simulink model "etc_ref"  (R2023a)
settings: Solver=ode45  StartTime=0.0  StopTime=20.0  RelTol=1e-3
PreLoadFcn:
  | etc_all_data;
undefined symbols (not defined in the file): J, Ki, Kp, Ts, Vdrop, Vfree, Vopen, Vrise
Description:
  | This is my help
settings Model: ParamWorkspaceSource=ReferencedWorkspace  Creator=nicholas  LastModifiedBy=Administrator
settings SolverCC: AlgebraicLoopSolver=TrustRegion
settings DataIOCC: LimitDataPoints=on  SaveFormat=Array  SignalLoggingSaveFormat=ModelDataLogs  ReturnWorkspaceOutputs=off  SignalLoggingName=sigsOut
settings OptimizationCC: InitFltsAndDblsToZero=on  LifeSpan=inf
settings DebuggingCC: SaveWithParameterizedLinksMsg=none  UnderspecifiedInitializationDetection=Classic  MergeDetectMultiDrivingBlocksExec=none  SignalResolutionControl=TryResolveAllWithWarning  MultiTaskDSMMsg=warning  MultiTaskCondExecSysMsg=none  FcnCallInpInsideContextMsg=warning  UnconnectedInputMsg=warning  UnconnectedOutputMsg=warning  UnconnectedLineMsg=warning  StateNameClashWarn=warning  SFUnexpectedBacktrackingDiag=warning  SFNoUnconditionalDefaultTransitionDiag=warning  SFExecutionAtInitializationDiag=none  ArithmeticOperatorsInVariantConditions=warning
settings HardwareCC: ProdBitPerPointer=32  ProdBitPerSizeT=32  ProdBitPerPtrDiffT=32  ProdLargestAtomicFloat=None  ProdIntDivRoundTo=Undefined  ProdEndianess=Unspecified  ProdWordSize=32  ProdHWDeviceType=32-bit Generic  TargetIntDivRoundTo=Zero  TargetEndianess=BigEndian  TargetHWDeviceType=Motorola PowerPC
settings ModelReferenceCC: PropagateSignalLabelsOutOfModel=off
settings SFSimCC: SimParseCustomCode=off
settings CodeAppCC: StateflowObjectComments=on
settings GRTTargetCC: TargetFcnLib=ansi_tfl_tmw.mat  TargetLangStandard=C89/C90 (ANSI)  CombineOutputUpdateFcns=off  GRTInterface=on
settings ConfigComp: CovMetricSettings=dw  CovSaveCumulativeToWorkspaceVar=on  CovSaveSingleToWorkspaceVar=on

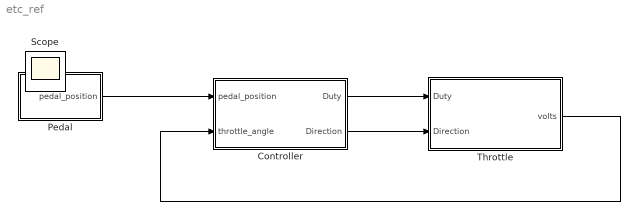
== system etc_ref ==
  Controller : Subsystem
  Pedal : Subsystem
  Throttle : Subsystem
  Scope : Scope
  wires:
  Pedal/1(pedal_position) -> Controller/1(pedal_position)
  Controller/1(Duty) -> Throttle/1(Duty)
  Controller/2(Direction) -> Throttle/2(Direction)
  Throttle/1(volts) -> Controller/2(throttle_angle)

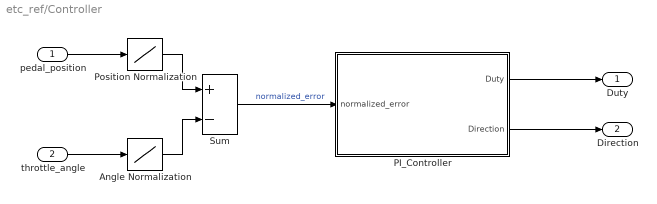
== system etc_ref/Controller ==
  pedal_position : Inport
  throttle_angle : Inport  Port=2
  Angle Normalization : Lookup  InputValues=[Vfree Vopen]  Table=[0 1]  LookUpMeth=Interpolation-Use End Values  SaturateOnIntegerOverflow=off
  PI_Controller : Subsystem
  Position Normalization : Lookup  InputValues=[Vdrop Vrise]  Table=[1 0]  LookUpMeth=Interpolation-Use End Values  SaturateOnIntegerOverflow=off
  Sum : Sum  Inputs=+-
  Duty : Outport
  Direction : Outport  Port=2
  wires:
  PI_Controller/2(Direction) -> Direction/1
  Position Normalization/1 -> Sum/1
  Angle Normalization/1 -> Sum/2
  Sum/1 -> PI_Controller/1(normalized_error)  "normalized_error"
  PI_Controller/1(Duty) -> Duty/1
  throttle_angle/1 -> Angle Normalization/1
  pedal_position/1 -> Position Normalization/1

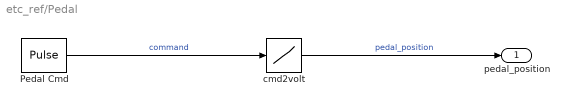
== system etc_ref/Pedal ==
  Pedal Cmd : DiscretePulseGenerator  PulseType=Time based  Amplitude=0.9  Period=10  PulseWidth=50  PhaseDelay=2.5
  cmd2volt : Lookup  InputValues=[0 1]  Table=[Vrise Vdrop]  LookUpMeth=Interpolation-Use End Values  SaturateOnIntegerOverflow=off
  pedal_position : Outport
  wires:
  Pedal Cmd/1 -> cmd2volt/1  "command"
  cmd2volt/1 -> pedal_position/1  "pedal_position"

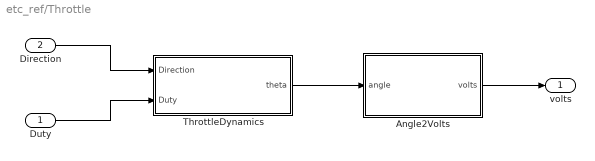
== system etc_ref/Throttle ==
  Duty : Inport
  Direction : Inport  Port=2
  Angle2Volts : Subsystem
  ThrottleDynamics : Subsystem
  volts : Outport
  wires:
  Angle2Volts/1(volts) -> volts/1
  ThrottleDynamics/1(theta) -> Angle2Volts/1("angle ")
  Duty/1 -> ThrottleDynamics/2(Duty)
  Direction/1 -> ThrottleDynamics/1(Direction)

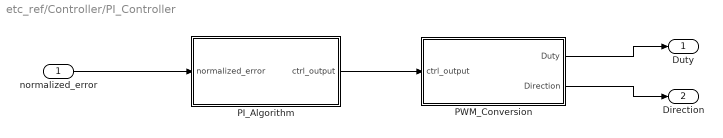
== system etc_ref/Controller/PI_Controller ==
  normalized_error : Inport  SampleTime=Ts
  PI_Algorithm : Subsystem
  PWM_Conversion : Subsystem
  Duty : Outport
  Direction : Outport  Port=2
  wires:
  PI_Algorithm/1(ctrl_output) -> PWM_Conversion/1(ctrl_output)
  PWM_Conversion/2(Direction) -> Direction/1
  PWM_Conversion/1("Duty ") -> Duty/1
  normalized_error/1 -> PI_Algorithm/1(normalized_error)

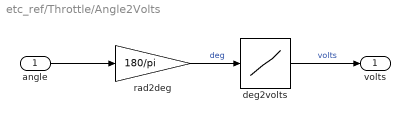
== system etc_ref/Throttle/Angle2Volts ==
  "angle " : Inport
  deg2volts : Lookup  InputValues=[0 90]  Table=[0.5 4.5]  SaturateOnIntegerOverflow=off
  rad2deg : Gain  Gain=180/pi  SaturateOnIntegerOverflow=on  OutDataTypeStr=Inherit: Same as input  ParamDataTypeStr=Inherit: Same as input
  volts : Outport
  wires:
  "angle "/1 -> rad2deg/1
  deg2volts/1 -> volts/1  "volts"
  rad2deg/1 -> deg2volts/1  "deg"

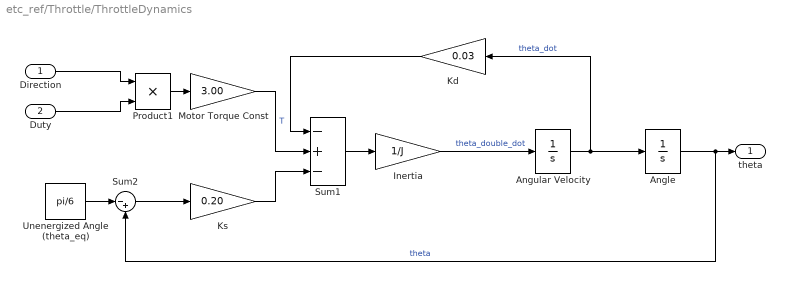
== system etc_ref/Throttle/ThrottleDynamics ==
  Direction : Inport
  Duty : Inport  Port=2
  Angle : Integrator  InitialCondition=pi/6  LimitOutput=on  UpperSaturationLimit=pi/2  LowerSaturationLimit=0
      settings: AttributesFormatString=Initial condition: %<InitialCondition>\n%<LowerSaturationLimit> <= theta <= %<UpperSaturationLimit>
  Angular Velocity : Integrator
      settings: AttributesFormatString=Initial condition: %<InitialCondition>
  Inertia : Gain  Gain=1/J  SaturateOnIntegerOverflow=on  OutDataTypeStr=Inherit: Same as input  ParamDataTypeStr=Inherit: Same as input
  Kd : Gain  Gain=0.03  SaturateOnIntegerOverflow=on  OutDataTypeStr=Inherit: Same as input  ParamDataTypeStr=Inherit: Same as input
  Ks : Gain  Gain=0.20  SaturateOnIntegerOverflow=on  OutDataTypeStr=Inherit: Same as input  ParamDataTypeStr=Inherit: Same as input
  Motor Torque Const : Gain  Gain=3.00  SaturateOnIntegerOverflow=on  OutDataTypeStr=Inherit: Same as input  ParamDataTypeStr=Inherit: Same as input
  Product1 : Product  SaturateOnIntegerOverflow=on  OutDataTypeStr=Inherit: Same as first input
  Sum1 : Sum  Inputs=-+-  SaturateOnIntegerOverflow=on
  Sum2 : Sum  Inputs=|-+  SaturateOnIntegerOverflow=on
  Unenergized Angle (theta_eq) : Constant  Value=pi/6
  theta : Outport
  wires:
  Sum1/1 -> Inertia/1
  Ks/1 -> Sum1/3
  Kd/1 -> Sum1/1
  Motor Torque Const/1 -> Sum1/2  "T"
  Duty/1 -> Product1/2
  Direction/1 -> Product1/1
  Inertia/1 -> Angular Velocity/1  "theta_double_dot"
  Angular Velocity/1 -> Kd/1, Angle/1  "theta_dot"
  Angle/1 -> theta/1, Sum2/2  "theta"
  Sum2/1 -> Ks/1
  Unenergized Angle (theta_eq)/1 -> Sum2/1
  Product1/1 -> Motor Torque Const/1

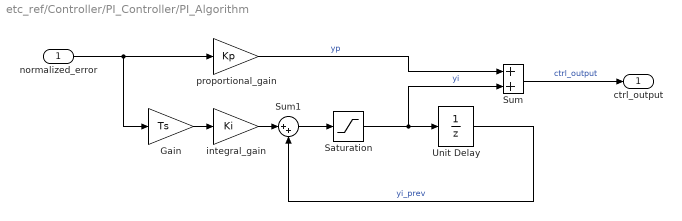
== system etc_ref/Controller/PI_Controller/PI_Algorithm ==
  normalized_error : Inport  SampleTime=Ts
      settings: AttributesFormatString=Sample time = %<SampleTime>
  Gain : Gain  Gain=Ts  SaturateOnIntegerOverflow=on  OutDataTypeStr=Inherit: Same as input  ParamDataTypeStr=Inherit: Same as input
  Saturation : Saturate  UpperLimit=1  LowerLimit=-1
      settings: AttributesFormatString=Max: %<UpperLimit>\nMin: %<LowerLimit>
  Sum : Sum  InputSameDT=on  SaturateOnIntegerOverflow=on  OutDataTypeStr=Inherit: Same as first input
  Sum1 : Sum  Inputs=|++  InputSameDT=on  SaturateOnIntegerOverflow=on  OutDataTypeStr=Inherit: Same as first input
  Unit Delay : UnitDelay  SampleTime=Ts
      settings: AttributesFormatString=yi0 = %<X0>\nSample time = %<SampleTime>
  integral_gain : Gain  Gain=Ki  SaturateOnIntegerOverflow=on  OutDataTypeStr=Inherit: Same as input  ParamDataTypeStr=Inherit: Same as input
  proportional_gain : Gain  Gain=Kp  SaturateOnIntegerOverflow=on  OutDataTypeStr=Inherit: Same as input  ParamDataTypeStr=Inherit: Same as input
  ctrl_output : Outport
  wires:
  Sum/1 -> ctrl_output/1  "ctrl_output"
  normalized_error/1 -> Gain/1, proportional_gain/1
  Saturation/1 -> Sum/2, Unit Delay/1  "yi"
  Sum1/1 -> Saturation/1
  Unit Delay/1 -> Sum1/2  "yi_prev"
  Gain/1 -> integral_gain/1
  integral_gain/1 -> Sum1/1
  proportional_gain/1 -> Sum/1  "yp"

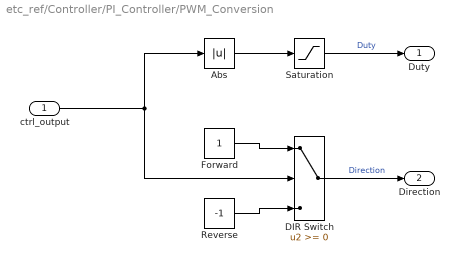
== system etc_ref/Controller/PI_Controller/PWM_Conversion ==
  ctrl_output : Inport
  Abs : Abs  SaturateOnIntegerOverflow=off
  DIR Switch : Switch  SaturateOnIntegerOverflow=off  InputSameDT=off
      settings: AttributesFormatString=Criteria: %<Criteria>\nThreshold: %<Threshold>
  Forward : Constant  OutDataTypeStr=double
  Reverse : Constant  Value=-1  OutDataTypeStr=double
  Saturation : Saturate  UpperLimit=1  LowerLimit=0
      settings: AttributesFormatString=%<LowerLimit> < duty < %<UpperLimit>
  "Duty " : Outport
  Direction : Outport  Port=2
  wires:
  ctrl_output/1 -> Abs/1, DIR Switch/2
  Forward/1 -> DIR Switch/1
  Reverse/1 -> DIR Switch/3
  DIR Switch/1 -> Direction/1  "Direction"
  Saturation/1 -> "Duty "/1  "Duty"
  Abs/1 -> Saturation/1
